simulink model "MODEL_NL"  (R2019a)
settings: Solver=VariableStepAuto  StartTime=0.0  StopTime=10.0  RelTol=1e-3
undefined symbols (not defined in the file or in its folder): g, LL, RR
settings Model: Creator=gaul2525  LastModifiedBy=gaul2525

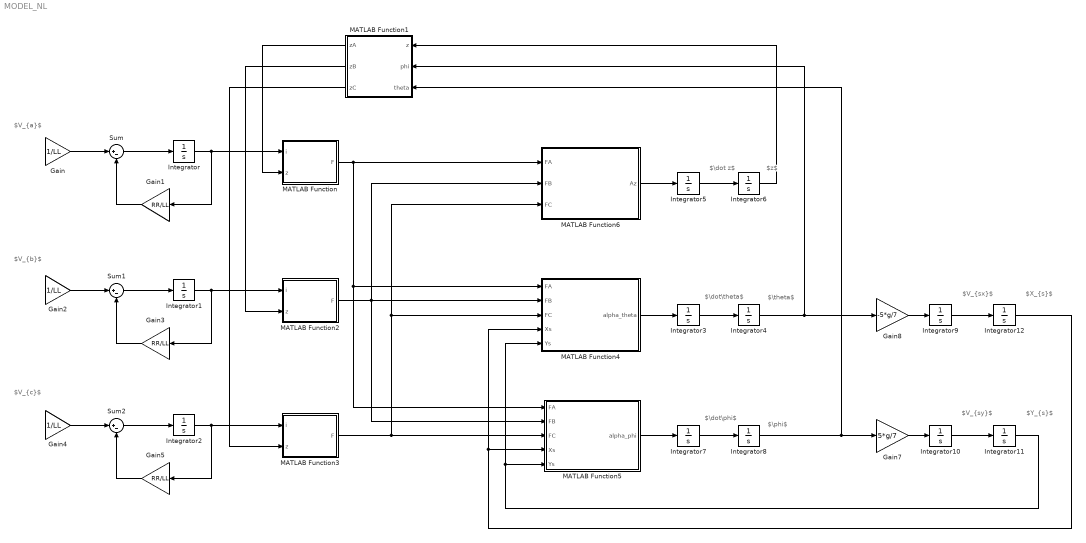
== system MODEL_NL ==
  note: $\theta$
  note: $\phi$
  note: $\dot\phi$
  note: $V_{sy}$
  note: $V_{sx}$
  note: $z$
  note: $\dot z$
  note: $\dot\theta$
  note: $X_{s}$
  note: $Y_{s}$
  note: $V_{a}$
  note: $V_{b}$
  note: $V_{c}$
  Gain : Gain  Gain=1/LL
  Gain1 : Gain  Gain=RR/LL
  Gain2 : Gain  Gain=1/LL
  Gain3 : Gain  Gain=RR/LL
  Gain4 : Gain  Gain=1/LL
  Gain5 : Gain  Gain=RR/LL
  Gain7 : Gain  Gain=5*g/7
  Gain8 : Gain  Gain=-5*g/7
  Integrator{,1..12} (13 alike) : Integrator
  MATLAB Function : MATLAB Function  TreatAsAtomicUnit=on
  MATLAB Function1 : MATLAB Function  TreatAsAtomicUnit=on
  MATLAB Function2 : MATLAB Function  TreatAsAtomicUnit=on
  MATLAB Function3 : MATLAB Function  TreatAsAtomicUnit=on
  MATLAB Function4 : MATLAB Function  TreatAsAtomicUnit=on
  MATLAB Function5 : MATLAB Function  TreatAsAtomicUnit=on
  MATLAB Function6 : MATLAB Function  TreatAsAtomicUnit=on
  Sum : Sum  Inputs=|+-
  Sum1 : Sum  Inputs=|+-
  Sum2 : Sum  Inputs=|+-
  wires:
  Gain/1 -> Sum/1
  Sum/1 -> Integrator/1
  Integrator/1 -> MATLAB Function/1(i), Gain1/1
  Gain1/1 -> Sum/2
  MATLAB Function1/1(zA) -> MATLAB Function/2(z)
  MATLAB Function1/2(zB) -> MATLAB Function2/2(z)
  MATLAB Function1/3(zC) -> MATLAB Function3/2(z)
  MATLAB Function/1(F) -> MATLAB Function6/1(FA), MATLAB Function4/1(FA), MATLAB Function5/1(FA)
  MATLAB Function2/1(F) -> MATLAB Function4/2(FB), MATLAB Function5/2(FB), MATLAB Function6/2(FB)
  MATLAB Function3/1(F) -> MATLAB Function5/3(FC), MATLAB Function4/3(FC), MATLAB Function6/3(FC)
  MATLAB Function4/1(alpha_theta) -> Integrator3/1
  Integrator3/1 -> Integrator4/1
  Integrator5/1 -> Integrator6/1
  Integrator7/1 -> Integrator8/1
  MATLAB Function5/1(alpha_phi) -> Integrator7/1
  Integrator6/1 -> MATLAB Function1/1(z)
  Integrator4/1 -> Gain8/1, MATLAB Function1/2(phi)
  Integrator8/1 -> Gain7/1, MATLAB Function1/3(theta)
  Gain8/1 -> Integrator9/1
  Gain7/1 -> Integrator10/1
  Integrator9/1 -> Integrator12/1
  Integrator10/1 -> Integrator11/1
  Integrator11/1 -> MATLAB Function4/5(Ys), MATLAB Function5/5(Ys)
  Integrator12/1 -> MATLAB Function4/4(Xs), MATLAB Function5/4(Xs)
  MATLAB Function6/1(Az) -> Integrator5/1
  Gain3/1 -> Sum1/2
  Gain2/1 -> Sum1/1
  Sum1/1 -> Integrator1/1
  Integrator1/1 -> MATLAB Function2/1(i), Gain3/1
  Gain5/1 -> Sum2/2
  Gain4/1 -> Sum2/1
  Sum2/1 -> Integrator2/1
  Integrator2/1 -> MATLAB Function3/1(i), Gain5/1

== matlab function MODEL_NL/MATLAB Function1 ==
  data: z input; phi input; zA output; theta input; zB output; zC output
function [zA,zB,zC] = fcn(z , phi , theta)

    zA = Z - Xa*theta + Ya*phi;
    
    zB = Z - Xb*theta + Yb*phi
    
    zC = Z - Xc*theta + Yc*phi

== matlab function MODEL_NL/MATLAB Function ==
  data: i input; F output; z input
function F = fcn(i , z)

    FSK = -1/(as0 + as1*z + as2*z^2 +as3*z^3);
    
    FEK = ((i^2 + be1*abs(i))*sign(i))/(ae0 + ae1*z + ae2*z^2 +ae3*z^3)

    F = FEK + FSK;

== matlab function MODEL_NL/MATLAB Function2 ==
  data: i input; F output; z input
function F = fcn(i , z)

    FSK = -1/(as0 + as1*z + as2*z^2 +as3*z^3);
    
    FEK = ((i^2 + be1*abs(i))*sign(i))/(ae0 + ae1*z + ae2*z^2 +ae3*z^3)

    F = FEK + FSK;

== matlab function MODEL_NL/MATLAB Function3 ==
  data: i input; F output; z input
function F = fcn(i , z)

    FSK = -1/(as0 + as1*z + as2*z^2 +as3*z^3);
    
    FEK = ((i^2 + be1*abs(i))*sign(i))/(ae0 + ae1*z + ae2*z^2 +ae3*z^3)

    F = FEK + FSK;

== matlab function MODEL_NL/MATLAB Function4 ==
  data: FA input; alpha_theta output; FB input; FC input; Xs input; Ys input; J parameter
function alpha_theta = fcn(FA , FB , FC, Xs , Ys, J)

    alpha_theta = (1/J)*(-FA*YA - FB*YB - FC*YC - Fs*Ys);

== matlab function MODEL_NL/MATLAB Function5 ==
  data: FA input; alpha_phi output; FB input; FC input; Xs input; Ys input
function alpha_phi = fcn(FA , FB , FC, Xs , Ys)

    alpha_phi = (1/J)*(FA*XA + FB*XB +FC*XC + Xs*Fs);

== matlab function MODEL_NL/MATLAB Function6 ==
  data: FA input; Az output; FB input; FC input
function Az = fcn(FA , FB , FC)

    Az = (FA + FB + FC + Fs)/m;
